simulink model "SynGen_Feedback_FieldVoltage"  (R2021b)
settings: Solver=VariableStepAuto  StartTime=0.0  StopTime=50  RelTol=1e-3
libraries: simulink x2, spsRMSLib x1, dspstat3 x1, spsSynchronousMachineSIFundamentalLib x1, spsThreePhaseParallelRLCLoadLib x1, spsThreePhaseVIMeasurementLib x1, spspowerguiLib x1
settings Model: Creator=User  LastModifiedBy=Tanvir Rahman

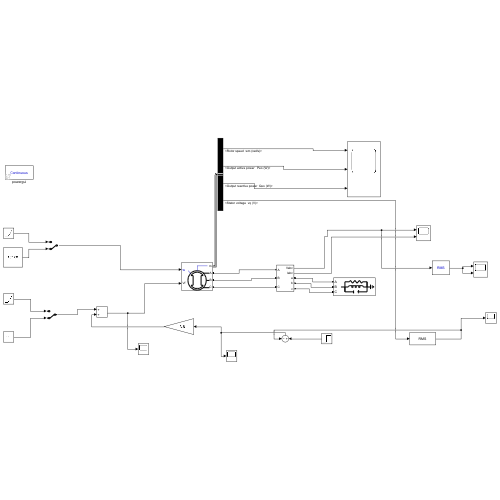
[thumbnail: Simulink's stored preview of the top-level diagram]
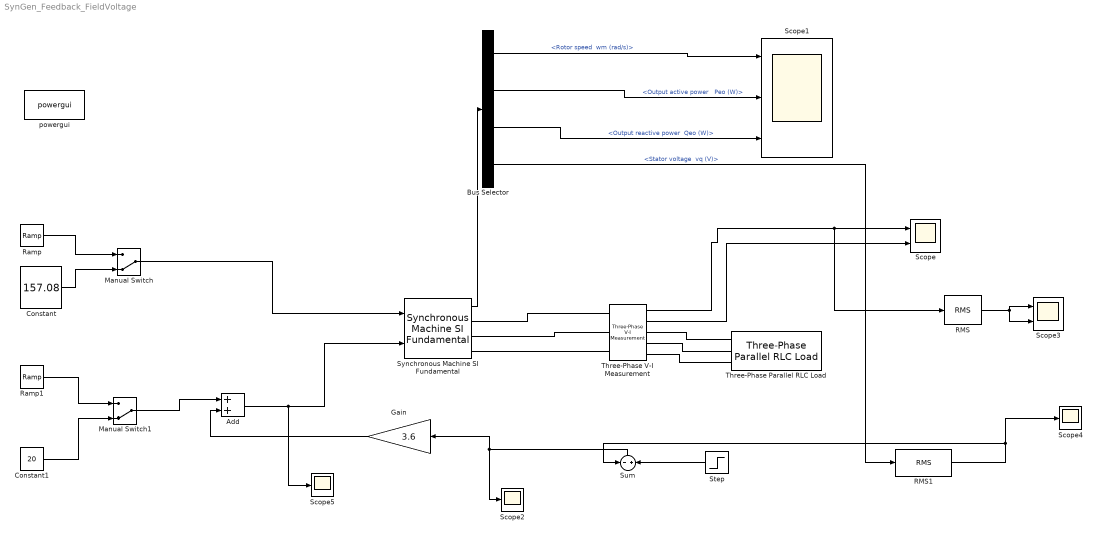
== system SynGen_Feedback_FieldVoltage ==
  Add : Sum
  Bus Selector : BusSelector  OutputSignals="Mechanical.Rotor speed  wm (rad/s),Output active power   Peo (W),Output reactive power  Qeo (W),dq0 components.Stator voltage  vq (V)"
  Constant : Constant  Value=157.08
  Constant1 : Constant  Value=20
  Gain : Gain  Gain=3.6
  Manual Switch : ManualSwitch  CurrentSetting=0
  Manual Switch1 : ManualSwitch  CurrentSetting=0
  RMS : spsRMSLib/RMS  TrueRMS=on  Freq=60  RMSInit=120  Ts=0
  RMS1 : dspstat3/RMS  run=off  directionMode=Each column  dimension=1  InputProcessing=Columns as channels (frame based)  reset_popup=None
  Ramp : simulink/Sources/Ramp  slope=1  start=0  InitialOutput=0
  Ramp1 : simulink/Sources/Ramp  slope=1  start=0  InitialOutput=0
  Scope : Scope  NumInputPorts=2
  Scope1 : Scope  NumInputPorts=3
  Scope2 : Scope
  Scope3 : Scope  NumInputPorts=2
  Scope4 : Scope
  Scope5 : Scope
  Step : Step  After=385.3  SampleTime=0
  Sum : Sum  Inputs=-+
  Synchronous Machine SI Fundamental : spsSynchronousMachineSIFundamentalLib/Synchronous Machine SI Fundamental  PresetModel=No  MechanicalLoad=Speed w  ShowDetailedParameters=on  RotorType=Salient-pole  Units=SI fundamental parameters  MeasurementBus=off  NominalParameters="[ 10e4  440   60   5 ]"  Stator="[ 2.9069E-03  3.0892E-04  3.2164E-03  9.7153E-04 ]"  Field="[ 5.9013E-04  3.0712E-04 ]"  Dampers2=[ 0.0664, 1.387e-3, 0.0292, 6.896e-4, 7.907e-3, 2.477e-3]  Dampers1="[ 1.1900E-02  4.9076E-04  2.0081E-02  1.0365E-03 ]"  Mechanical=[ 3.895e6 0 20 ]  PolePairs=2  InitialConditions="[ 0  0  0  0  0  0  0  0  70.3192 ]"  SetSaturation=off  Saturation=[695.64,774.7,917.5,1001.6,1082.2,1175.9,1293.6,1430.2,1583.7;9660,10623,12243,13063,13757,14437,15180,15890,16567]  DisplayVfd=off  LoadFlowParameters=[1,0,0,0,0]  TsPowergui=0  TsBlock=-1  IterativeModel=Trapezoidal non iterative  IterativeDiscreteModel=Trapezoidal non iterative  BusType=PV  Pref=0  Qref=0  Qmin=-inf  Qmax=inf  PLF=0  QLF=0
      settings: SourceProductBaseCode=PS
  Three-Phase Parallel RLC Load : spsThreePhaseParallelRLCLoadLib/Three-Phase Parallel RLC Load  LConnTagsString=A|B|C  Configuration=Y (grounded)  NominalVoltage=440  Vabc=[1e3 1e3 1e3]  Vabcp=[1e3 1e3 1e3]  NominalFrequency=60  UnbalancedPower=off  ActivePower=1  InductivePower=1  CapacitivePower=1  Pabc=[10e3 9e3 11e3]  QLabc=[100 90 110]  QCabc=[100 90 110]  Pabcp=[10e3 9e3 11e3]  QLabcp=[100 90 110]  QCabcp=[100 90 110]  Measurements=None  LoadType=constant Z
  Three-Phase V-I Measurement : spsThreePhaseVIMeasurementLib/Three-Phase V-I Measurement  VoltageMeasurement=phase-to-ground  SetLabelV=off  LabelV=Vabc  Vpu=off  VpuLL=off  CurrentMeasurement=yes  SetLabelI=off  LabelI=Iabc  Ipu=off  Pbase=100e6  Vbase=500e3  OutputType=Complex  PhasorSimulation=off  PSBequivalent=0
  powergui : spspowerguiLib/powergui  Priority=1  SimulationMode=Continuous  SampleTime=50e-6  frequency=60  Iterations=50  frequencyindice=60  Pbase=100e6  ErrMax=1e-4  UnitsV=kV  UnitsW=MW  buscounter=0  FunctionMessages=off  echomessages=off  EnableUseOfTLC=off  CurrentSourceSwitches=off  DisableSnubberDevices=off  DisableRonSwitches=off  DisableVfSwitches=off  DisplayEquations=off  AutomaticDiscreteSolvers=off  SolverType=Tustin/Backward Euler (TBE)  Interpol=off  ExternalGateDelay=off  methode=off  Ts=100  x0status=blocks  SPID=on  SwTol=0  HookPort=off  NonlinearTolerance=1e-4  nMaxIteration=100  ContinueOnMaxIteration=off  RestoreLinks=warning  ResistiveCurrentMeasurement=off  Frange=[0:2:500]  Ylog=off  Xlog=on  ShowGrid=off  save=off  variable=ZData  structure=0  ZoomFFT=off  StartTime=0.0  cycles=1  DisplayStyle=1  fundamental=60  FreqAxis=off  MaxFrequency=1000  frequencyindicesteady=1  RmsSteady=1  display=off
  wires:
  Ramp/1 -> Manual Switch/1
  Constant/1 -> Manual Switch/2
  Ramp1/1 -> Manual Switch1/1
  Constant1/1 -> Manual Switch1/2
  Three-Phase V-I Measurement/2 -> Scope/2
  Synchronous Machine SI Fundamental/1 -> Bus Selector/1
  Bus Selector/1 -> Scope1/1  "<Rotor speed  wm (rad/s)>"
  Bus Selector/2 -> Scope1/2  "<Output active power   Peo (W)>"
  Bus Selector/3 -> Scope1/3  "<Output reactive power  Qeo (W)>"
  Three-Phase V-I Measurement/1 -> RMS/1, Scope/1
  RMS/1 -> Scope3/1, Scope3/2
  Bus Selector/4 -> RMS1/1  "<Stator voltage  vq (V)>"
  RMS1/1 -> Scope4/1, Sum/1
  Step/1 -> Sum/2
  Sum/1 -> Scope2/1, Gain/1
  Manual Switch1/1 -> Add/1
  Gain/1 -> Add/2
  Add/1 -> Scope5/1, Synchronous Machine SI Fundamental/2
  Manual Switch/1 -> Synchronous Machine SI Fundamental/1
  connections:
  Synchronous Machine SI Fundamental/RConn1 -- Three-Phase V-I Measurement/LConn1
  Synchronous Machine SI Fundamental/RConn2 -- Three-Phase V-I Measurement/LConn2
  Synchronous Machine SI Fundamental/RConn3 -- Three-Phase V-I Measurement/LConn3
  Three-Phase V-I Measurement/RConn1 -- Three-Phase Parallel RLC Load/LConn1
  Three-Phase V-I Measurement/RConn2 -- Three-Phase Parallel RLC Load/LConn2
  Three-Phase Parallel RLC Load/LConn3 -- Three-Phase V-I Measurement/RConn3
